simulink model "Rocket"  (R2021a)
settings: Solver=VariableStepAuto  StartTime=0.0  StopTime=600  MaxStep=0.1  RelTol=1e-3
libraries: simulink x2, simulink_extras x1
settings Model: Creator=honor  LastModifiedBy=Gleb
settings SolverCC: AlgebraicLoopSolver=TrustRegion
settings DebuggingCC: SFMachineParentedDataDiag=warning

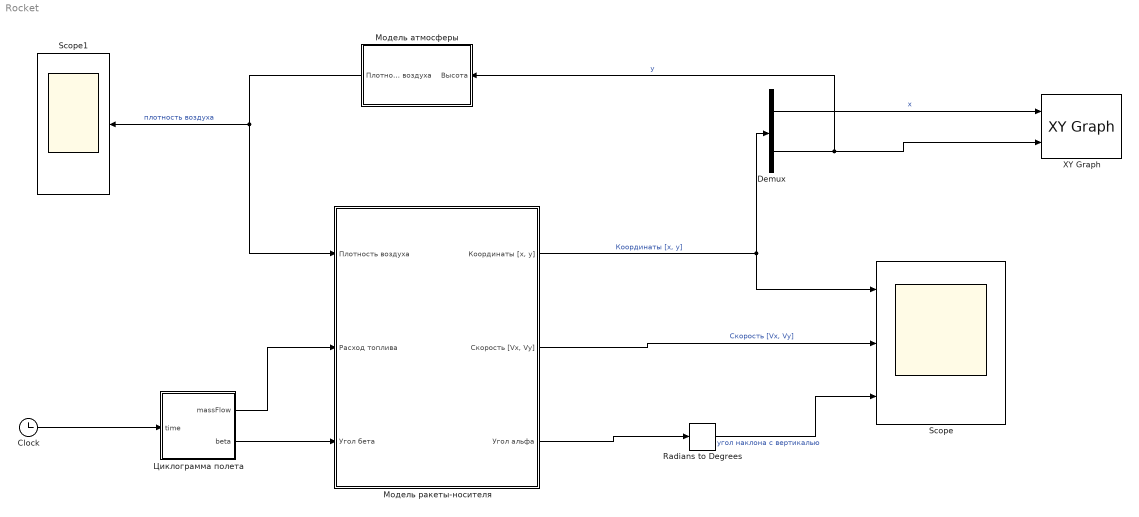
== system Rocket ==
  Clock : Clock
  Demux : Demux  Outputs=2
  Radians to Degrees : simulink_extras/Transformations/Radians to Degrees
  Scope : Scope  NumInputPorts=3
  Scope1 : Scope
  XY Graph : simulink/Sinks/XY Graph  xmin=-1  xmax=3e6  ymin=-1  ymax=1e6  st=-1
  Модель атмосферы : Subsystem  mask{M=0.029, R=8.31, g=9.81, T=300, P0=1}
      mask prompts: M "молярная масса воздуха"; R "универскальная газовая постоянная"; g "ускорение свободного падения"; T "температура"; P0 "плотность на высоте 0 метров"
  Модель ракеты-носителя : Subsystem  mask{L=70, Mr=1e4, Mt=1e4, S=10, g=9.8}
      mask prompts: L "длина ракеты (м)"; Mr "Масса незаправленной ракеты (кг)"; Mt "Стартовая масса топлива (кг)"; S "Площадь сечения ракеты (м^2)"; g "Ускорение свободного падения"
  Циклограмма полета : MATLAB Function  TreatAsAtomicUnit=on
  wires:
  Clock/1 -> Циклограмма полета/1(time)
  Циклограмма полета/1(massFlow) -> Модель ракеты-носителя/2(Расход топлива)
  Циклограмма полета/2(beta) -> Модель ракеты-носителя/3(Угол бета)
  Модель ракеты-носителя/3(Угол альфа) -> Radians to Degrees/1
  Radians to Degrees/1 -> Scope/3  "угол наклона с вертикалью"
  Модель ракеты-носителя/2("Скорость [Vx, Vy]") -> Scope/2  "Скорость [Vx, Vy]"
  Модель ракеты-носителя/1("Координаты [x, y]") -> Demux/1, Scope/1  "Координаты [x, y]"
  Модель атмосферы/1(Плотность воздуха) -> Модель ракеты-носителя/1(Плотность воздуха), Scope1/1  "плотность воздуха"
  Demux/1 -> XY Graph/1  "x"
  Demux/2 -> XY Graph/2, Модель атмосферы/1(Высота)  "y"

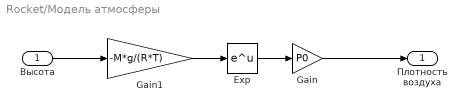
== system Rocket/Модель атмосферы ==
  Высота : Inport
  Exp : Math  SaturateOnIntegerOverflow=on
  Gain : Gain  Gain=P0
  Gain1 : Gain  Gain=-M*g/(R*T)
  Плотность воздуха : Outport
  wires:
  Exp/1 -> Gain/1
  Gain/1 -> Плотность воздуха/1
  Высота/1 -> Gain1/1
  Gain1/1 -> Exp/1

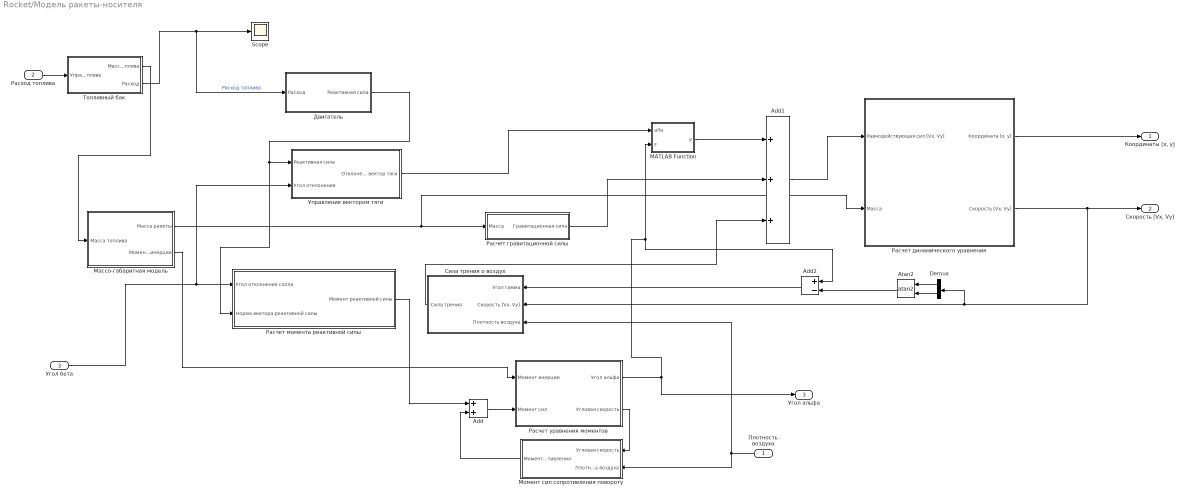
== system Rocket/Модель ракеты-носителя ==
  Плотность воздуха : Inport
  Расход топлива : Inport  Port=2
  Угол бета : Inport  Port=3
  Add : Sum
  Add1 : Sum  Inputs=+++
  Add2 : Sum  Inputs=+-
  Atan2 : Trigonometry  Operator=atan2
  Demux : Demux  Outputs=2
  MATLAB Function : MATLAB Function  TreatAsAtomicUnit=on
  Scope : Scope
  Двигатель : Subsystem  mask{dv=2e4}
      mask prompts: dv "Скорость истечения газов (м/c)"
  Массо-габаритная модель : Subsystem
  Момент сил сопротивления повороту : Subsystem
  Расчет гравитационной силы : Subsystem
  Расчет динамического уравнения : Subsystem
  Расчет момента реактивной силы : Subsystem
  Расчет уравнения моментов : Subsystem
  Сила трения о воздух : Subsystem
  Топливный бак : Subsystem
  Управление вектором тяги : Subsystem
  "Координаты [x, y]" : Outport
  "Скорость [Vx, Vy]" : Outport  Port=2
  Угол альфа : Outport  Port=3
  wires:
  Расход топлива/1 -> Топливный бак/1(Управление расходом топлива)
  Топливный бак/1("Масса топлива ") -> Массо-габаритная модель/1(Масса топлива)
  Массо-габаритная модель/1(Масса ракеты) -> Расчет динамического уравнения/2(Масса), Расчет гравитационной силы/1("Масса ")
  Топливный бак/2(Расход) -> Scope/1, Двигатель/1(Расход)  "Расход топлива"
  Двигатель/1(Реактивная сила) -> Расчет момента реактивной силы/2(Норма вектора реактивной силы), Управление вектором тяги/1(Реактивная сила)
  Угол бета/1 -> Управление вектором тяги/2(Угол отклонения), Расчет момента реактивной силы/1(Угол отклонения сопла)
  Расчет момента реактивной силы/1(Момент реактивной силы) -> Add/1
  Add/1 -> Расчет уравнения моментов/2(Момент сил)
  Массо-габаритная модель/2(Момент инерции) -> Расчет уравнения моментов/1(Момент инерции)
  Момент сил сопротивления повороту/1(Момент сопротивления) -> Add/2
  Расчет уравнения моментов/2(Угловая скорость) -> Момент сил сопротивления повороту/1(Угловая скорость)
  Расчет уравнения моментов/1(Угол альфа) -> Угол альфа/1, Add2/1, MATLAB Function/2(F)
  Плотность воздуха/1 -> Сила трения о воздух/3(Плотность воздуха), Момент сил сопротивления повороту/2(Плотность воздуха)
  Сила трения о воздух/1(Сила трения) -> Add1/3
  Расчет гравитационной силы/1(Гравитационная сила) -> Add1/2
  MATLAB Function/1(y) -> Add1/1
  Расчет динамического уравнения/1("Координата [x, y]") -> "Координаты [x, y]"/1
  Расчет динамического уравнения/2("Скорость [Vx, Vy]") -> Сила трения о воздух/2("Скорость [Vx, Vy]"), Demux/1, "Скорость [Vx, Vy]"/1
  Add1/1 -> Расчет динамического уравнения/1("Равнодействующая сил [Vx, Vy]")
  Demux/1 -> Atan2/1
  Demux/2 -> Atan2/2
  Add2/1 -> Сила трения о воздух/1(Угол гамма)
  Atan2/1 -> Add2/2
  Управление вектором тяги/1(Отклоненный вектор тяги) -> MATLAB Function/1(alfa)

== system Rocket/Модель ракеты-носителя/Двигатель ==
  Расход : Inport
  Gain : Gain  Gain=dv
  Реактивная сила : Outport
  wires:
  Gain/1 -> Реактивная сила/1
  Расход/1 -> Gain/1

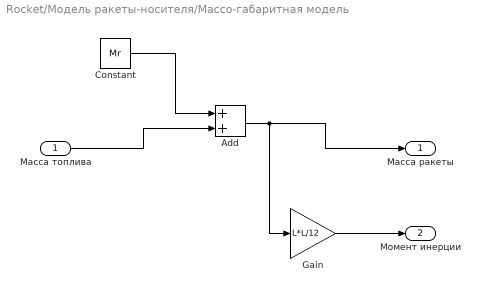
== system Rocket/Модель ракеты-носителя/Массо-габаритная модель ==
  Масса топлива : Inport
  Add : Sum
  Constant : Constant  Value=Mr
  Gain : Gain  Gain=L*L/12
  Масса ракеты : Outport
  Момент инерции : Outport  Port=2
  wires:
  Масса топлива/1 -> Add/2
  Add/1 -> Gain/1, Масса ракеты/1
  Constant/1 -> Add/1
  Gain/1 -> Момент инерции/1

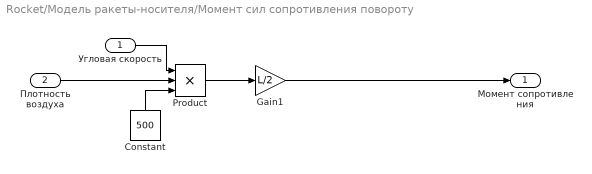
== system Rocket/Модель ракеты-носителя/Момент сил сопротивления повороту ==
  Угловая скорость : Inport
  Плотность воздуха : Inport  Port=2
  Constant : Constant  Value=500
  Gain1 : Gain  Gain=L/2
  Product : Product  Inputs=3
  Момент сопротивления : Outport
  wires:
  Плотность воздуха/1 -> Product/2
  Угловая скорость/1 -> Product/1
  Constant/1 -> Product/3
  Product/1 -> Gain1/1
  Gain1/1 -> Момент сопротивления/1

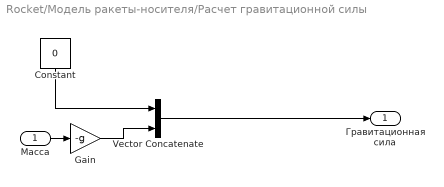
== system Rocket/Модель ракеты-носителя/Расчет гравитационной силы ==
  "Масса " : Inport
  Constant : Constant  Value=0
  Gain : Gain  Gain=-g
  Vector Concatenate : Concatenate
  Гравитационная сила : Outport
  wires:
  "Масса "/1 -> Gain/1
  Vector Concatenate/1 -> Гравитационная сила/1
  Gain/1 -> Vector Concatenate/2
  Constant/1 -> Vector Concatenate/1

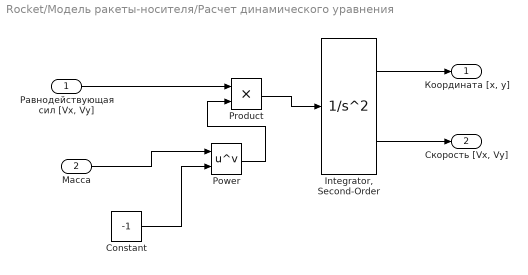
== system Rocket/Модель ракеты-носителя/Расчет динамического уравнения ==
  "Равнодействующая сил [Vx, Vy]" : Inport
  Масса : Inport  Port=2
  Constant : Constant  Value=-1
  "Integrator, Second-Order" : SecondOrderIntegrator
  Power : Math  Operator=pow  SaturateOnIntegerOverflow=on
  Product : Product
  "Координата [x, y]" : Outport
  "Скорость [Vx, Vy]" : Outport  Port=2
  wires:
  "Integrator, Second-Order"/1 -> "Координата [x, y]"/1
  "Integrator, Second-Order"/2 -> "Скорость [Vx, Vy]"/1
  Масса/1 -> Power/1
  Constant/1 -> Power/2
  "Равнодействующая сил [Vx, Vy]"/1 -> Product/1
  Power/1 -> Product/2
  Product/1 -> "Integrator, Second-Order"/1

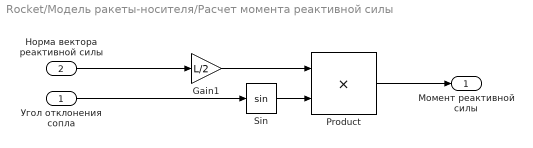
== system Rocket/Модель ракеты-носителя/Расчет момента реактивной силы ==
  Угол отклонения сопла : Inport
  Норма вектора реактивной силы : Inport  Port=2
  Gain1 : Gain  Gain=L/2
  Product : Product
  Sin : Trigonometry
  Момент реактивной силы : Outport
  wires:
  Норма вектора реактивной силы/1 -> Gain1/1
  Угол отклонения сопла/1 -> Sin/1
  Gain1/1 -> Product/1
  Sin/1 -> Product/2
  Product/1 -> Момент реактивной силы/1

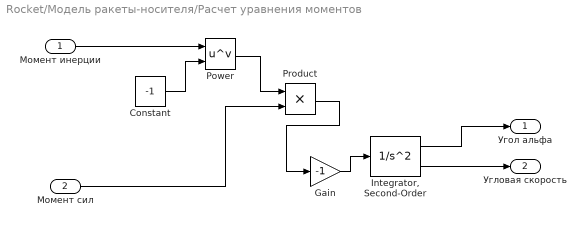
== system Rocket/Модель ракеты-носителя/Расчет уравнения моментов ==
  Момент инерции : Inport
  Момент сил : Inport  Port=2
  Constant : Constant  Value=-1
  Gain : Gain  Gain=-1
  "Integrator, Second-Order" : SecondOrderIntegrator
  Power : Math  Operator=pow  SaturateOnIntegerOverflow=on
  Product : Product
  Угол альфа : Outport
  Угловая скорость : Outport  Port=2
  wires:
  Power/1 -> Product/1
  Момент сил/1 -> Product/2
  Product/1 -> Gain/1
  "Integrator, Second-Order"/2 -> Угловая скорость/1
  "Integrator, Second-Order"/1 -> Угол альфа/1
  Constant/1 -> Power/2
  Момент инерции/1 -> Power/1
  Gain/1 -> "Integrator, Second-Order"/1

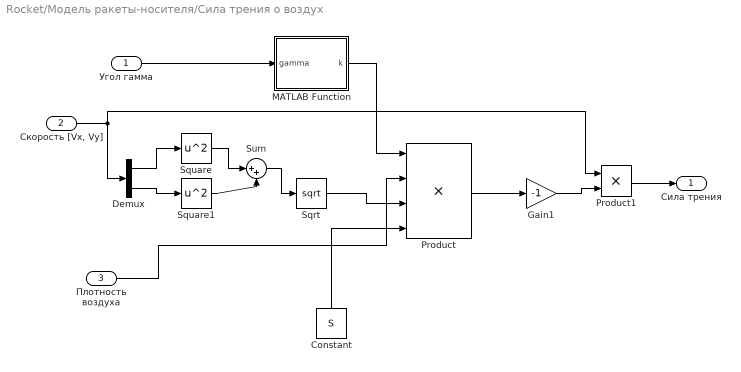
== system Rocket/Модель ракеты-носителя/Сила трения о воздух ==
  Угол гамма : Inport
  "Скорость [Vx, Vy]" : Inport  Port=2
  Плотность воздуха : Inport  Port=3
  Constant : Constant  Value=S
  Demux : Demux  Outputs=2
  Gain1 : Gain  Gain=-1
  MATLAB Function : MATLAB Function  TreatAsAtomicUnit=on
  Product : Product  Inputs=4
  Product1 : Product
  Sqrt : Sqrt  SaturateOnIntegerOverflow=on
  Square : Math  Operator=square  SaturateOnIntegerOverflow=on
  Square1 : Math  Operator=square  SaturateOnIntegerOverflow=on
  Sum : Sum  Inputs=|++
  Сила трения : Outport
  wires:
  Угол гамма/1 -> MATLAB Function/1(gamma)
  MATLAB Function/1(k) -> Product/1
  "Скорость [Vx, Vy]"/1 -> Product1/1, Demux/1
  Demux/1 -> Square/1
  Demux/2 -> Square1/1
  Square/1 -> Sum/1
  Square1/1 -> Sum/2
  Constant/1 -> Product/4
  Плотность воздуха/1 -> Product/2
  Sum/1 -> Sqrt/1
  Sqrt/1 -> Product/3
  Product/1 -> Gain1/1
  Product1/1 -> Сила трения/1
  Gain1/1 -> Product1/2

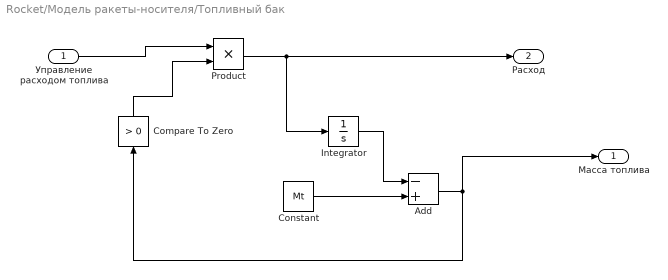
== system Rocket/Модель ракеты-носителя/Топливный бак ==
  Управление расходом топлива : Inport
  Add : Sum  Inputs=-+
  Compare To Zero : simulink/Logic and Bit Operations/Compare To Zero  relop=>  OutDataTypeStr=boolean
  Constant : Constant  Value=Mt
  Integrator : Integrator
  Product : Product
  "Масса топлива " : Outport
  Расход : Outport  Port=2
  wires:
  Управление расходом топлива/1 -> Product/1
  Compare To Zero/1 -> Product/2
  Product/1 -> Integrator/1, Расход/1
  Integrator/1 -> Add/1
  Constant/1 -> Add/2
  Add/1 -> Compare To Zero/1, "Масса топлива "/1

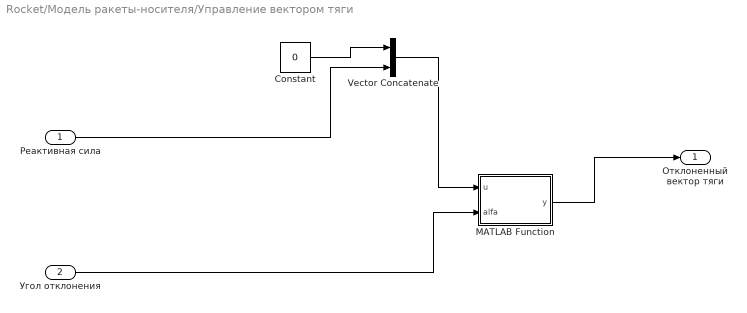
== system Rocket/Модель ракеты-носителя/Управление вектором тяги ==
  Реактивная сила : Inport
  Угол отклонения : Inport  Port=2
  Constant : Constant  Value=0
  MATLAB Function : MATLAB Function  TreatAsAtomicUnit=on
  Vector Concatenate : Concatenate
  Отклоненный вектор тяги : Outport
  wires:
  MATLAB Function/1(y) -> Отклоненный вектор тяги/1
  Реактивная сила/1 -> Vector Concatenate/2
  Constant/1 -> Vector Concatenate/1
  Vector Concatenate/1 -> MATLAB Function/1(u)
  Угол отклонения/1 -> MATLAB Function/2(alfa)

== matlab function Rocket/Модель ракеты-носителя/MATLAB Function ==
  data: alfa input; F input; y output
function y = fcn(alfa, F)
S = [cos(F) sin(F); -sin(F) cos(F)];
y = S * alfa;

== matlab function Rocket/Циклограмма полета ==
  data: time input; massFlow output; beta output
function [massFlow, beta] = fcn(time)
if time < 80
    beta = 0;
elseif time < 120
    beta = -0.0001;
elseif time < 200
    beta = 0;
elseif time < 240
    beta = 0.00007;
else
    beta = 0;
end
massFlow = 20;

== matlab function Rocket/Модель ракеты-носителя/Сила трения о воздух/MATLAB Function ==
  data: gamma input; k output
function k = fcn(gamma)
gamma(gamma > pi) = 2 * pi - gamma(gamma > pi);
if (gamma <= pi/8)
    k = 1;
elseif (gamma > 7 * pi/8)
    k = 2;
else
    k = 10;
end

== matlab function Rocket/Модель ракеты-носителя/Управление вектором тяги/MATLAB Function ==
  data: u input; y output; alfa input
function y  = fcn(u, alfa)
A = [cos(alfa) sin(alfa); -sin(alfa) cos(alfa)];
y = A * u;
